simulink model "test_version"  (R2022b)
settings: Solver=VariableStepAuto  StartTime=0.0  StopTime=10.0  RelTol=1e-3
libraries: fl_lib x8, nesl_utility x2, ee_lib x1
settings Model: Creator=lenovo  LastModifiedBy=lenovo

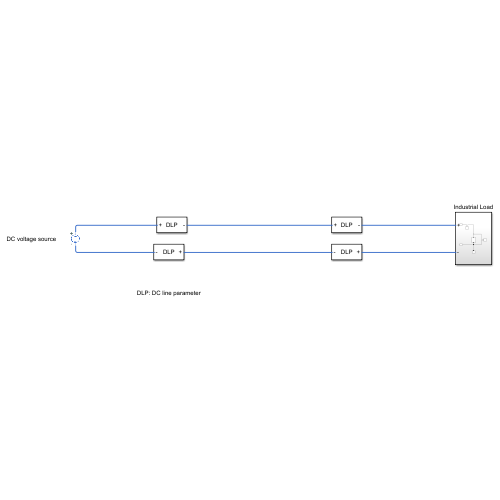
[thumbnail: Simulink's stored preview of the top-level diagram]
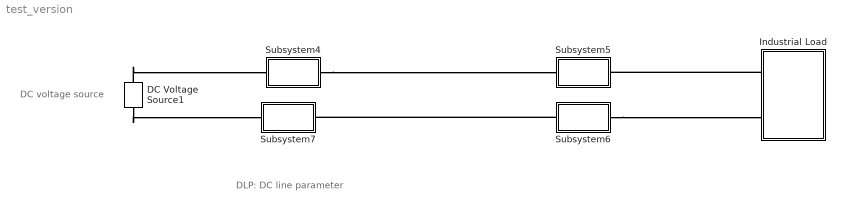
== system test_version ==
  note: DC voltage source
  note: DLP: DC line parameter
  DC Voltage Source1 : ee_lib/Additional Components/SPICE Sources/DC Voltage Source  DC=12 V
  Industrial Load : Subsystem
  Subsystem4 : Subsystem
      mask Display:
      | disp('DLP')
      | port_label('LConn',1,'+')
      | port_label('RConn',1,'-')
  Subsystem5 : Subsystem
      mask Display:
      | disp('DLP')
      | port_label('LConn',1,'+')
      | port_label('RConn',1,'-')
  Subsystem6 : Subsystem
      mask Display:
      | disp('DLP')
      | port_label('LConn',1,'+')
      | port_label('RConn',1,'-')
  Subsystem7 : Subsystem
      mask Display:
      | disp('DLP')
      | port_label('LConn',1,'+')
      | port_label('RConn',1,'-')
  connections:
  Subsystem4/RConn1 -- Subsystem5/LConn1
  Subsystem6/RConn1 -- Subsystem7/LConn1
  DC Voltage Source1/LConn1 -- Subsystem4/LConn1
  DC Voltage Source1/RConn1 -- Subsystem7/RConn1
  Industrial Load/LConn1 -- Subsystem5/RConn1
  Subsystem6/LConn1 -- Industrial Load/LConn2

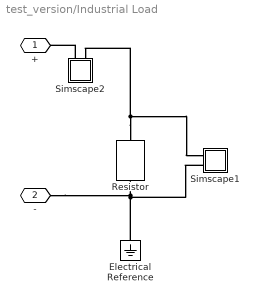
== system test_version/Industrial Load ==
  Electrical Reference : fl_lib/Electrical/Electrical Elements/Electrical Reference
  Resistor : fl_lib/Electrical/Electrical Elements/Resistor  R=1 Ohm  i_specify=off  i_priority=None  i=0 A  i_nominal_specify=off  i_nominal_unit=A  i_nominal_value=1  v_specify=off  v_priority=None  v=0 V  v_nominal_specify=off  v_nominal_unit=V  v_nominal_value=1
  Simscape1 : Subsystem
      mask Display:
      | disp('V')
      | port_label('LConn',1,'+')
      | port_label('LConn',2,'-')
  Simscape2 : Subsystem
      mask Display:
      | disp('A')
      | port_label('LConn',1,'+')
      | port_label('LConn',2,'-')
  + : PMIOPort  Side=Left
  - : PMIOPort  Port=2  Side=Left
  connections:
  Electrical Reference/LConn1 -- -/RConn1 -- Resistor/RConn1 -- Simscape1/LConn2
  Resistor/LConn1 -- Simscape2/LConn2 -- Simscape1/LConn1
  Simscape2/LConn1 -- +/RConn1

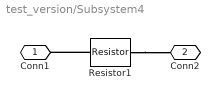
== system test_version/Subsystem4 ==
  Resistor1 : fl_lib/Electrical/Electrical Elements/Resistor  R=1 Ohm  i_specify=off  i_priority=None  i=0 A  i_nominal_specify=off  i_nominal_unit=A  i_nominal_value=1  v_specify=off  v_priority=None  v=0 V  v_nominal_specify=off  v_nominal_unit=V  v_nominal_value=1
  Conn1 : PMIOPort  Side=Left
  Conn2 : PMIOPort  Port=2  Side=Right
  connections:
  Resistor1/LConn1 -- Conn1/RConn1
  Resistor1/RConn1 -- Conn2/RConn1

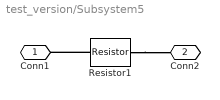
== system test_version/Subsystem5 ==
  Resistor1 : fl_lib/Electrical/Electrical Elements/Resistor  R=1 Ohm  i_specify=off  i_priority=None  i=0 A  i_nominal_specify=off  i_nominal_unit=A  i_nominal_value=1  v_specify=off  v_priority=None  v=0 V  v_nominal_specify=off  v_nominal_unit=V  v_nominal_value=1
  Conn1 : PMIOPort  Side=Left
  Conn2 : PMIOPort  Port=2  Side=Right
  connections:
  Resistor1/RConn1 -- Conn2/RConn1
  Resistor1/LConn1 -- Conn1/RConn1

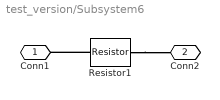
== system test_version/Subsystem6 ==
  Resistor1 : fl_lib/Electrical/Electrical Elements/Resistor  R=1 Ohm  i_specify=off  i_priority=None  i=0 A  i_nominal_specify=off  i_nominal_unit=A  i_nominal_value=1  v_specify=off  v_priority=None  v=0 V  v_nominal_specify=off  v_nominal_unit=V  v_nominal_value=1
  Conn1 : PMIOPort  Side=Left
  Conn2 : PMIOPort  Port=2  Side=Right
  connections:
  Resistor1/LConn1 -- Conn1/RConn1
  Resistor1/RConn1 -- Conn2/RConn1

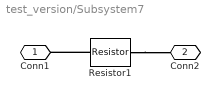
== system test_version/Subsystem7 ==
  Resistor1 : fl_lib/Electrical/Electrical Elements/Resistor  R=1 Ohm  i_specify=off  i_priority=None  i=0 A  i_nominal_specify=off  i_nominal_unit=A  i_nominal_value=1  v_specify=off  v_priority=None  v=0 V  v_nominal_specify=off  v_nominal_unit=V  v_nominal_value=1
  Conn1 : PMIOPort  Side=Left
  Conn2 : PMIOPort  Port=2  Side=Right
  connections:
  Resistor1/RConn1 -- Conn2/RConn1
  Resistor1/LConn1 -- Conn1/RConn1

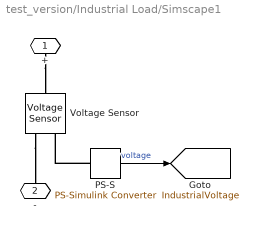
== system test_version/Industrial Load/Simscape1 ==
  PS-S : nesl_utility/PS-Simulink Converter  PhysicalDomain=network_engine_domain  SubClassName=ps_output  LeftPortType=input  RightPortType=output  PseudoPeriodic=off  Frequencies=[]  VectorFormat=1-D array  Unit=V  AffineConversion=off
  Voltage Sensor : fl_lib/Electrical/Electrical Sensors/Voltage Sensor
  + : PMIOPort  Side=Left
  - : PMIOPort  Port=2  Side=Left
  tag scope: IndustrialVoltage=global
  wires:
  PS-S/1 -> [IndustrialVoltage]  "voltage"
  connections:
  Voltage Sensor/RConn2 -- -/RConn1
  +/RConn1 -- Voltage Sensor/LConn1
  PS-S/LConn1 -- Voltage Sensor/RConn1

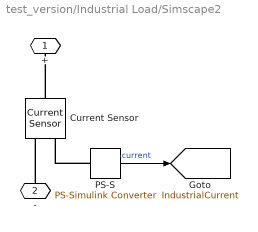
== system test_version/Industrial Load/Simscape2 ==
  Current Sensor : fl_lib/Electrical/Electrical Sensors/Current Sensor
  PS-S : nesl_utility/PS-Simulink Converter  PhysicalDomain=network_engine_domain  SubClassName=ps_output  LeftPortType=input  RightPortType=output  PseudoPeriodic=off  Frequencies=[]  VectorFormat=1-D array  Unit=A  AffineConversion=off
  + : PMIOPort  Side=Left
  - : PMIOPort  Port=2  Side=Left
  tag scope: IndustrialCurrent=global
  wires:
  PS-S/1 -> [IndustrialCurrent]  "current"
  connections:
  PS-S/LConn1 -- Current Sensor/RConn1
  Current Sensor/LConn1 -- +/RConn1
  -/RConn1 -- Current Sensor/RConn2
